simulink model "Appl_DrMemory_CtrlModel"  (R2018b)
settings: configuration reference "CodeConfig_10_ms" (kept outside this file)
undefined symbols (not defined in the file): CAL_DrMem_100MS, CAL_DrMem_90MS, D_DRMEM_SPEED_5, D_ToleranceDistance, FALSE, TRUE
libraries: DareLib x92, simulink x1
(part 2 of 3)

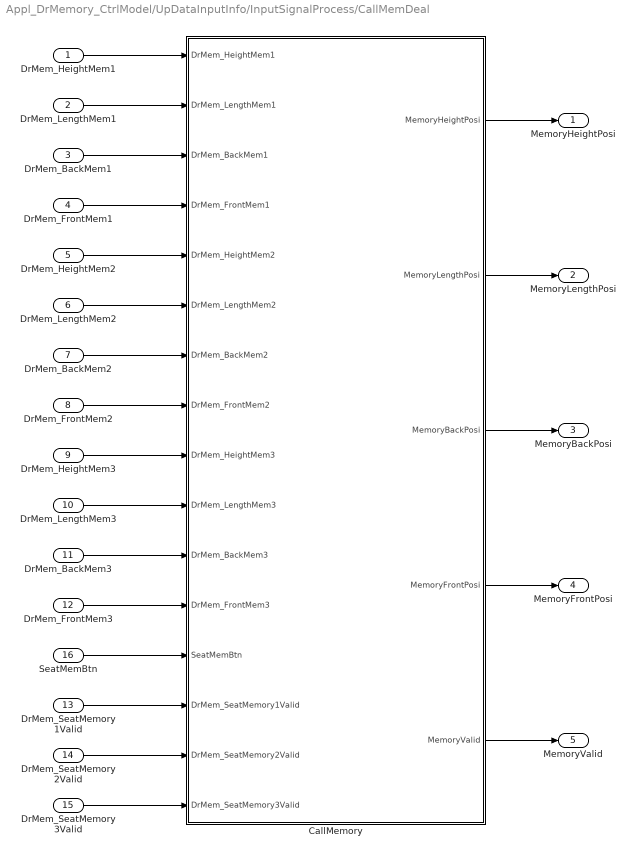
== system Appl_DrMemory_CtrlModel/UpDataInputInfo/InputSignalProcess/CallMemDeal ==
  DrMem_HeightMem1 : Inport
  DrMem_LengthMem1 : Inport  Port=2
  DrMem_BackMem1 : Inport  Port=3
  DrMem_FrontMem1 : Inport  Port=4
  DrMem_HeightMem2 : Inport  Port=5
  DrMem_LengthMem2 : Inport  Port=6
  DrMem_BackMem2 : Inport  Port=7
  DrMem_FrontMem2 : Inport  Port=8
  DrMem_HeightMem3 : Inport  Port=9
  DrMem_LengthMem3 : Inport  Port=10
  DrMem_BackMem3 : Inport  Port=11
  DrMem_FrontMem3 : Inport  Port=12
  DrMem_SeatMemory1Valid : Inport  Port=13
  DrMem_SeatMemory2Valid : Inport  Port=14
  DrMem_SeatMemory3Valid : Inport  Port=15
  SeatMemBtn : Inport  Port=16
  CallMemory : Stateflow chart  TreatAsAtomicUnit=on
  MemoryHeightPosi : Outport
  MemoryLengthPosi : Outport  Port=2
  MemoryBackPosi : Outport  Port=3
  MemoryFrontPosi : Outport  Port=4
  MemoryValid : Outport  Port=5
  wires:
  DrMem_LengthMem1/1 -> CallMemory/2(DrMem_LengthMem1)
  DrMem_BackMem1/1 -> CallMemory/3(DrMem_BackMem1)
  DrMem_HeightMem1/1 -> CallMemory/1(DrMem_HeightMem1)
  DrMem_FrontMem1/1 -> CallMemory/4(DrMem_FrontMem1)
  DrMem_HeightMem2/1 -> CallMemory/5(DrMem_HeightMem2)
  DrMem_LengthMem2/1 -> CallMemory/6(DrMem_LengthMem2)
  DrMem_BackMem2/1 -> CallMemory/7(DrMem_BackMem2)
  DrMem_FrontMem2/1 -> CallMemory/8(DrMem_FrontMem2)
  DrMem_HeightMem3/1 -> CallMemory/9(DrMem_HeightMem3)
  DrMem_LengthMem3/1 -> CallMemory/10(DrMem_LengthMem3)
  DrMem_BackMem3/1 -> CallMemory/11(DrMem_BackMem3)
  SeatMemBtn/1 -> CallMemory/13(SeatMemBtn)
  DrMem_FrontMem3/1 -> CallMemory/12(DrMem_FrontMem3)
  CallMemory/1(MemoryHeightPosi) -> MemoryHeightPosi/1
  CallMemory/3(MemoryBackPosi) -> MemoryBackPosi/1
  CallMemory/4(MemoryFrontPosi) -> MemoryFrontPosi/1
  CallMemory/2(MemoryLengthPosi) -> MemoryLengthPosi/1
  CallMemory/5(MemoryValid) -> MemoryValid/1
  DrMem_SeatMemory3Valid/1 -> CallMemory/16(DrMem_SeatMemory3Valid)
  DrMem_SeatMemory2Valid/1 -> CallMemory/15(DrMem_SeatMemory2Valid)
  DrMem_SeatMemory1Valid/1 -> CallMemory/14(DrMem_SeatMemory1Valid)

== system Appl_DrMemory_CtrlModel/UpDataInputInfo/InputSignalProcess/HmiMessageDeal ==
  DrMem_IVI_FLSeatMemSet1 : Inport
  DrMem_IVI_FLSeatMemSet2 : Inport  Port=2
  DrMem_IVI_FLSeatMemSet3 : Inport  Port=3
  HmiDeal : Stateflow chart  TreatAsAtomicUnit=on
  SeatMemBtn : Outport
  wires:
  DrMem_IVI_FLSeatMemSet1/1 -> HmiDeal/1(DrMem_IVI_FLSeatMemSet1)
  DrMem_IVI_FLSeatMemSet2/1 -> HmiDeal/2(DrMem_IVI_FLSeatMemSet2)
  HmiDeal/1(SeatMemBtn) -> SeatMemBtn/1
  DrMem_IVI_FLSeatMemSet3/1 -> HmiDeal/3(DrMem_IVI_FLSeatMemSet3)

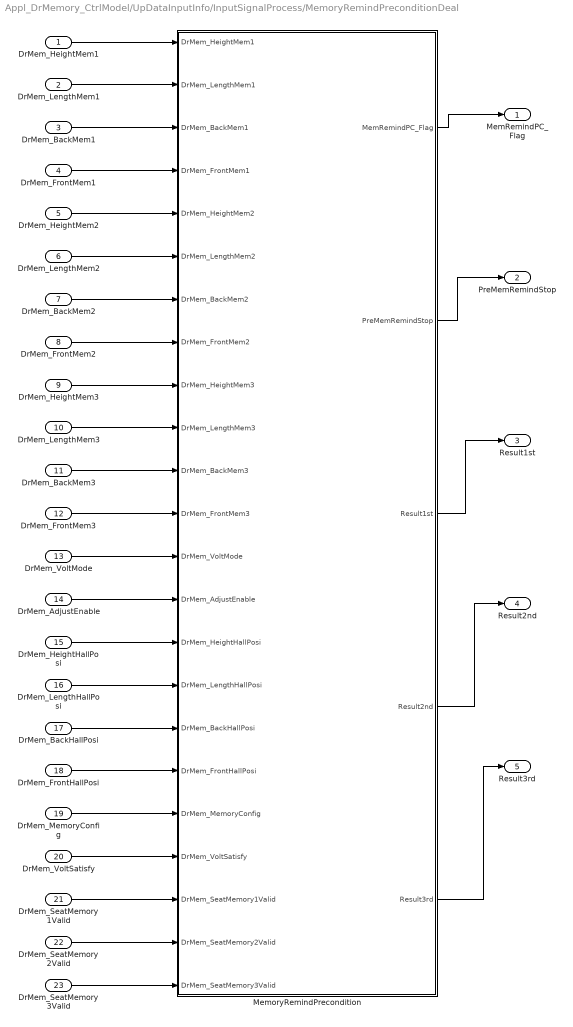
== system Appl_DrMemory_CtrlModel/UpDataInputInfo/InputSignalProcess/MemoryRemindPreconditionDeal ==
  DrMem_HeightMem1 : Inport
  DrMem_LengthMem1 : Inport  Port=2
  DrMem_BackMem1 : Inport  Port=3
  DrMem_FrontMem1 : Inport  Port=4
  DrMem_HeightMem2 : Inport  Port=5
  DrMem_LengthMem2 : Inport  Port=6
  DrMem_BackMem2 : Inport  Port=7
  DrMem_FrontMem2 : Inport  Port=8
  DrMem_HeightMem3 : Inport  Port=9
  DrMem_LengthMem3 : Inport  Port=10
  DrMem_BackMem3 : Inport  Port=11
  DrMem_FrontMem3 : Inport  Port=12
  DrMem_VoltMode : Inport  Port=13
  DrMem_AdjustEnable : Inport  Port=14
  DrMem_HeightHallPosi : Inport  Port=15
  DrMem_LengthHallPosi : Inport  Port=16
  DrMem_BackHallPosi : Inport  Port=17
  DrMem_FrontHallPosi : Inport  Port=18
  DrMem_MemoryConfig : Inport  Port=19
  DrMem_VoltSatisfy : Inport  Port=20
  DrMem_SeatMemory1Valid : Inport  Port=21
  DrMem_SeatMemory2Valid : Inport  Port=22
  DrMem_SeatMemory3Valid : Inport  Port=23
  MemoryRemindPrecondition : Stateflow chart  TreatAsAtomicUnit=on
  MemRemindPC_Flag : Outport
  PreMemRemindStop : Outport  Port=2
  Result1st : Outport  Port=3
  Result2nd : Outport  Port=4
  Result3rd : Outport  Port=5
  wires:
  DrMem_FrontMem3/1 -> MemoryRemindPrecondition/12(DrMem_FrontMem3)
  DrMem_VoltMode/1 -> MemoryRemindPrecondition/13(DrMem_VoltMode)
  DrMem_BackMem3/1 -> MemoryRemindPrecondition/11(DrMem_BackMem3)
  DrMem_LengthMem3/1 -> MemoryRemindPrecondition/10(DrMem_LengthMem3)
  DrMem_HeightMem3/1 -> MemoryRemindPrecondition/9(DrMem_HeightMem3)
  DrMem_FrontMem2/1 -> MemoryRemindPrecondition/8(DrMem_FrontMem2)
  DrMem_BackMem2/1 -> MemoryRemindPrecondition/7(DrMem_BackMem2)
  DrMem_LengthMem2/1 -> MemoryRemindPrecondition/6(DrMem_LengthMem2)
  DrMem_HeightMem2/1 -> MemoryRemindPrecondition/5(DrMem_HeightMem2)
  DrMem_FrontMem1/1 -> MemoryRemindPrecondition/4(DrMem_FrontMem1)
  DrMem_HeightMem1/1 -> MemoryRemindPrecondition/1(DrMem_HeightMem1)
  DrMem_BackMem1/1 -> MemoryRemindPrecondition/3(DrMem_BackMem1)
  DrMem_LengthMem1/1 -> MemoryRemindPrecondition/2(DrMem_LengthMem1)
  DrMem_AdjustEnable/1 -> MemoryRemindPrecondition/14(DrMem_AdjustEnable)
  DrMem_HeightHallPosi/1 -> MemoryRemindPrecondition/15(DrMem_HeightHallPosi)
  DrMem_LengthHallPosi/1 -> MemoryRemindPrecondition/16(DrMem_LengthHallPosi)
  DrMem_BackHallPosi/1 -> MemoryRemindPrecondition/17(DrMem_BackHallPosi)
  DrMem_FrontHallPosi/1 -> MemoryRemindPrecondition/18(DrMem_FrontHallPosi)
  MemoryRemindPrecondition/1(MemRemindPC_Flag) -> MemRemindPC_Flag/1
  MemoryRemindPrecondition/2(PreMemRemindStop) -> PreMemRemindStop/1
  MemoryRemindPrecondition/3(Result1st) -> Result1st/1
  MemoryRemindPrecondition/4(Result2nd) -> Result2nd/1
  MemoryRemindPrecondition/5(Result3rd) -> Result3rd/1
  DrMem_MemoryConfig/1 -> MemoryRemindPrecondition/19(DrMem_MemoryConfig)
  DrMem_VoltSatisfy/1 -> MemoryRemindPrecondition/20(DrMem_VoltSatisfy)
  DrMem_SeatMemory1Valid/1 -> MemoryRemindPrecondition/21(DrMem_SeatMemory1Valid)
  DrMem_SeatMemory3Valid/1 -> MemoryRemindPrecondition/23(DrMem_SeatMemory3Valid)
  DrMem_SeatMemory2Valid/1 -> MemoryRemindPrecondition/22(DrMem_SeatMemory2Valid)

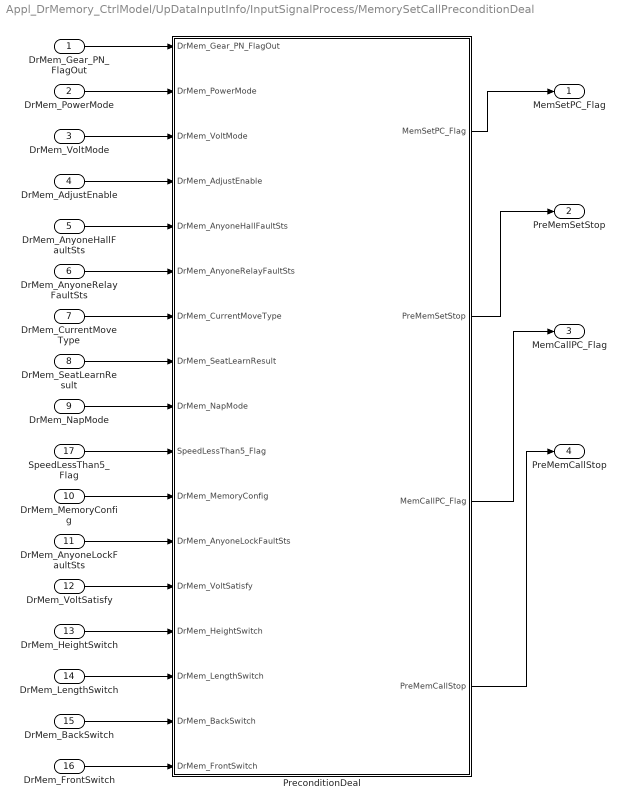
== system Appl_DrMemory_CtrlModel/UpDataInputInfo/InputSignalProcess/MemorySetCallPreconditionDeal ==
  DrMem_Gear_PN_FlagOut : Inport
  DrMem_PowerMode : Inport  Port=2
  DrMem_VoltMode : Inport  Port=3
  DrMem_AdjustEnable : Inport  Port=4
  DrMem_AnyoneHallFaultSts : Inport  Port=5
  DrMem_AnyoneRelayFaultSts : Inport  Port=6
  DrMem_CurrentMoveType : Inport  Port=7
  DrMem_SeatLearnResult : Inport  Port=8
  DrMem_NapMode : Inport  Port=9
  DrMem_MemoryConfig : Inport  Port=10
  DrMem_AnyoneLockFaultSts : Inport  Port=11
  DrMem_VoltSatisfy : Inport  Port=12
  DrMem_HeightSwitch : Inport  Port=13
  DrMem_LengthSwitch : Inport  Port=14
  DrMem_BackSwitch : Inport  Port=15
  DrMem_FrontSwitch : Inport  Port=16
  SpeedLessThan5_Flag : Inport  Port=17
  PreconditionDeal : Stateflow chart  TreatAsAtomicUnit=on
  MemSetPC_Flag : Outport
  PreMemSetStop : Outport  Port=2
  MemCallPC_Flag : Outport  Port=3
  PreMemCallStop : Outport  Port=4
  wires:
  DrMem_Gear_PN_FlagOut/1 -> PreconditionDeal/1(DrMem_Gear_PN_FlagOut)
  DrMem_PowerMode/1 -> PreconditionDeal/2(DrMem_PowerMode)
  DrMem_VoltMode/1 -> PreconditionDeal/3(DrMem_VoltMode)
  DrMem_AdjustEnable/1 -> PreconditionDeal/4(DrMem_AdjustEnable)
  DrMem_AnyoneHallFaultSts/1 -> PreconditionDeal/5(DrMem_AnyoneHallFaultSts)
  DrMem_CurrentMoveType/1 -> PreconditionDeal/7(DrMem_CurrentMoveType)
  DrMem_SeatLearnResult/1 -> PreconditionDeal/8(DrMem_SeatLearnResult)
  DrMem_NapMode/1 -> PreconditionDeal/9(DrMem_NapMode)
  SpeedLessThan5_Flag/1 -> PreconditionDeal/10(SpeedLessThan5_Flag)
  DrMem_AnyoneRelayFaultSts/1 -> PreconditionDeal/6(DrMem_AnyoneRelayFaultSts)
  PreconditionDeal/1(MemSetPC_Flag) -> MemSetPC_Flag/1
  PreconditionDeal/2(PreMemSetStop) -> PreMemSetStop/1
  PreconditionDeal/3(MemCallPC_Flag) -> MemCallPC_Flag/1
  PreconditionDeal/4(PreMemCallStop) -> PreMemCallStop/1
  DrMem_MemoryConfig/1 -> PreconditionDeal/11(DrMem_MemoryConfig)
  DrMem_AnyoneLockFaultSts/1 -> PreconditionDeal/12(DrMem_AnyoneLockFaultSts)
  DrMem_VoltSatisfy/1 -> PreconditionDeal/13(DrMem_VoltSatisfy)
  DrMem_HeightSwitch/1 -> PreconditionDeal/14(DrMem_HeightSwitch)
  DrMem_LengthSwitch/1 -> PreconditionDeal/15(DrMem_LengthSwitch)
  DrMem_BackSwitch/1 -> PreconditionDeal/16(DrMem_BackSwitch)
  DrMem_FrontSwitch/1 -> PreconditionDeal/17(DrMem_FrontSwitch)

== system Appl_DrMemory_CtrlModel/UpDataInputInfo/InputSignalProcess/VehicleSpeedDeal ==
  DrMem_0x284_SpeedLostFlag : Inport
  DrMem_VehicleSpeedValid : Inport  Port=2
  DrMem_VehicleSpeed : Inport  Port=3
  SpeedDeal : Stateflow chart  TreatAsAtomicUnit=on
  "SpeedLessThan5_Flag " : Outport
  wires:
  SpeedDeal/1(SpeedLessThan5_Flag) -> "SpeedLessThan5_Flag "/1
  DrMem_0x284_SpeedLostFlag/1 -> SpeedDeal/1(DrMem_0x284_SpeedLostFlag)
  DrMem_VehicleSpeedValid/1 -> SpeedDeal/2(DrMem_VehicleSpeedValid)
  DrMem_VehicleSpeed/1 -> SpeedDeal/3(DrMem_VehicleSpeed)

== system Appl_DrMemory_CtrlModel/LogicCtrl/LocalAdjustCtrl/MemorySetLogic/FirstPosiMemSetFunc/FirstPosiMemSetFunc/MemoryBack ==
  CurrentB : Inport
  f : TriggerPort  TriggerType=function-call  VariantControl=(inherit)
      settings: CopyFcn=Stateflow.SLINSF.SimulinkMan.removeBlockPreDeleteFcn  PreDeleteFcn=Stateflow.SLINSF.SimulinkMan.unsafePredeleteFcn
  WelcomeRunStatus : DareLib/Dare/setAPI_type  g_funcname=Srvl_SetMemIndexDataU16  g_param=EN_MemIndex_DrMem1_Back  g_type=uint16  g_size=-1
      settings: AttributesFormatString=%<g_funcname>  SourceProductName=Dare Library
  wires:
  CurrentB/1 -> WelcomeRunStatus/1

== system Appl_DrMemory_CtrlModel/LogicCtrl/LocalAdjustCtrl/MemorySetLogic/FirstPosiMemSetFunc/FirstPosiMemSetFunc/MemoryFront ==
  CurrentF : Inport
  f : TriggerPort  TriggerType=function-call  VariantControl=(inherit)
      settings: CopyFcn=Stateflow.SLINSF.SimulinkMan.removeBlockPreDeleteFcn  PreDeleteFcn=Stateflow.SLINSF.SimulinkMan.unsafePredeleteFcn
  WelcomeRunStatus : DareLib/Dare/setAPI_type  g_funcname=Srvl_SetMemIndexDataU16  g_param=EN_MemIndex_DrMem1_Front  g_type=uint16  g_size=-1
      settings: AttributesFormatString=%<g_funcname>  SourceProductName=Dare Library
  wires:
  CurrentF/1 -> WelcomeRunStatus/1

== system Appl_DrMemory_CtrlModel/LogicCtrl/LocalAdjustCtrl/MemorySetLogic/FirstPosiMemSetFunc/FirstPosiMemSetFunc/MemoryHight ==
  CurrentH : Inport
  f : TriggerPort  TriggerType=function-call  VariantControl=(inherit)
      settings: CopyFcn=Stateflow.SLINSF.SimulinkMan.removeBlockPreDeleteFcn  PreDeleteFcn=Stateflow.SLINSF.SimulinkMan.unsafePredeleteFcn
  WelcomeRunStatus : DareLib/Dare/setAPI_type  g_funcname=Srvl_SetMemIndexDataU16  g_param=EN_MemIndex_DrMem1_Height  g_type=uint16  g_size=-1
      settings: AttributesFormatString=%<g_funcname>  SourceProductName=Dare Library
  wires:
  CurrentH/1 -> WelcomeRunStatus/1

== system Appl_DrMemory_CtrlModel/LogicCtrl/LocalAdjustCtrl/MemorySetLogic/FirstPosiMemSetFunc/FirstPosiMemSetFunc/MemoryLength ==
  CurrentL : Inport
  f : TriggerPort  TriggerType=function-call  VariantControl=(inherit)
      settings: CopyFcn=Stateflow.SLINSF.SimulinkMan.removeBlockPreDeleteFcn  PreDeleteFcn=Stateflow.SLINSF.SimulinkMan.unsafePredeleteFcn
  WelcomeRunStatus : DareLib/Dare/setAPI_type  g_funcname=Srvl_SetMemIndexDataU16  g_param=EN_MemIndex_DrMem1_Length  g_type=uint16  g_size=-1
      settings: AttributesFormatString=%<g_funcname>  SourceProductName=Dare Library
  wires:
  CurrentL/1 -> WelcomeRunStatus/1

== system Appl_DrMemory_CtrlModel/LogicCtrl/LocalAdjustCtrl/MemorySetLogic/FirstPosiMemSetFunc/FirstPosiMemSetFunc/MemoryValid ==
  Sts : Inport
  f : TriggerPort  TriggerType=function-call  VariantControl=(inherit)
      settings: CopyFcn=Stateflow.SLINSF.SimulinkMan.removeBlockPreDeleteFcn  PreDeleteFcn=Stateflow.SLINSF.SimulinkMan.unsafePredeleteFcn
  WelcomeRunStatus : DareLib/Dare/setAPI_type  g_funcname=Srvl_SetMemIndexDataU8  g_param=EN_MemIndex_DrMem1_ValidFlag  g_type=uint16  g_size=-1
      settings: AttributesFormatString=%<g_funcname>  SourceProductName=Dare Library
  wires:
  Sts/1 -> WelcomeRunStatus/1

== system Appl_DrMemory_CtrlModel/LogicCtrl/LocalAdjustCtrl/MemorySetLogic/SecondPosiMemSetFunc/SecondPosiMemSetFunc/MemoryBack ==
  CurrentB : Inport
  f : TriggerPort  TriggerType=function-call  VariantControl=(inherit)
      settings: CopyFcn=Stateflow.SLINSF.SimulinkMan.removeBlockPreDeleteFcn  PreDeleteFcn=Stateflow.SLINSF.SimulinkMan.unsafePredeleteFcn
  WelcomeRunStatus : DareLib/Dare/setAPI_type  g_funcname=Srvl_SetMemIndexDataU16  g_param=EN_MemIndex_DrMem2_Back  g_type=uint16  g_size=-1
      settings: AttributesFormatString=%<g_funcname>  SourceProductName=Dare Library
  wires:
  CurrentB/1 -> WelcomeRunStatus/1

== system Appl_DrMemory_CtrlModel/LogicCtrl/LocalAdjustCtrl/MemorySetLogic/SecondPosiMemSetFunc/SecondPosiMemSetFunc/MemoryFront ==
  CurrentF : Inport
  f : TriggerPort  TriggerType=function-call  VariantControl=(inherit)
      settings: CopyFcn=Stateflow.SLINSF.SimulinkMan.removeBlockPreDeleteFcn  PreDeleteFcn=Stateflow.SLINSF.SimulinkMan.unsafePredeleteFcn
  WelcomeRunStatus : DareLib/Dare/setAPI_type  g_funcname=Srvl_SetMemIndexDataU16  g_param=EN_MemIndex_DrMem2_Front  g_type=uint16  g_size=-1
      settings: AttributesFormatString=%<g_funcname>  SourceProductName=Dare Library
  wires:
  CurrentF/1 -> WelcomeRunStatus/1

== system Appl_DrMemory_CtrlModel/LogicCtrl/LocalAdjustCtrl/MemorySetLogic/SecondPosiMemSetFunc/SecondPosiMemSetFunc/MemoryHight ==
  CurrentH : Inport
  f : TriggerPort  TriggerType=function-call  VariantControl=(inherit)
      settings: CopyFcn=Stateflow.SLINSF.SimulinkMan.removeBlockPreDeleteFcn  PreDeleteFcn=Stateflow.SLINSF.SimulinkMan.unsafePredeleteFcn
  WelcomeRunStatus : DareLib/Dare/setAPI_type  g_funcname=Srvl_SetMemIndexDataU16  g_param=EN_MemIndex_DrMem2_Height  g_type=uint16  g_size=-1
      settings: AttributesFormatString=%<g_funcname>  SourceProductName=Dare Library
  wires:
  CurrentH/1 -> WelcomeRunStatus/1

== system Appl_DrMemory_CtrlModel/LogicCtrl/LocalAdjustCtrl/MemorySetLogic/SecondPosiMemSetFunc/SecondPosiMemSetFunc/MemoryLength ==
  CurrentL : Inport
  f : TriggerPort  TriggerType=function-call  VariantControl=(inherit)
      settings: CopyFcn=Stateflow.SLINSF.SimulinkMan.removeBlockPreDeleteFcn  PreDeleteFcn=Stateflow.SLINSF.SimulinkMan.unsafePredeleteFcn
  WelcomeRunStatus : DareLib/Dare/setAPI_type  g_funcname=Srvl_SetMemIndexDataU16  g_param=EN_MemIndex_DrMem2_Length  g_type=uint16  g_size=-1
      settings: AttributesFormatString=%<g_funcname>  SourceProductName=Dare Library
  wires:
  CurrentL/1 -> WelcomeRunStatus/1

== system Appl_DrMemory_CtrlModel/LogicCtrl/LocalAdjustCtrl/MemorySetLogic/SecondPosiMemSetFunc/SecondPosiMemSetFunc/MemoryValid ==
  Sts : Inport
  f : TriggerPort  TriggerType=function-call  VariantControl=(inherit)
      settings: CopyFcn=Stateflow.SLINSF.SimulinkMan.removeBlockPreDeleteFcn  PreDeleteFcn=Stateflow.SLINSF.SimulinkMan.unsafePredeleteFcn
  WelcomeRunStatus : DareLib/Dare/setAPI_type  g_funcname=Srvl_SetMemIndexDataU8  g_param=EN_MemIndex_DrMem2_ValidFlag  g_type=uint16  g_size=-1
      settings: AttributesFormatString=%<g_funcname>  SourceProductName=Dare Library
  wires:
  Sts/1 -> WelcomeRunStatus/1

== system Appl_DrMemory_CtrlModel/LogicCtrl/LocalAdjustCtrl/MemorySetLogic/ThirdPosiMemSetFunc/ThirdPosiMemSetFunc/MemoryBack ==
  CurrentB : Inport
  f : TriggerPort  TriggerType=function-call  VariantControl=(inherit)
      settings: CopyFcn=Stateflow.SLINSF.SimulinkMan.removeBlockPreDeleteFcn  PreDeleteFcn=Stateflow.SLINSF.SimulinkMan.unsafePredeleteFcn
  WelcomeRunStatus : DareLib/Dare/setAPI_type  g_funcname=Srvl_SetMemIndexDataU16  g_param=EN_MemIndex_DrMem3_Back  g_type=uint16  g_size=-1
      settings: AttributesFormatString=%<g_funcname>  SourceProductName=Dare Library
  wires:
  CurrentB/1 -> WelcomeRunStatus/1

== system Appl_DrMemory_CtrlModel/LogicCtrl/LocalAdjustCtrl/MemorySetLogic/ThirdPosiMemSetFunc/ThirdPosiMemSetFunc/MemoryFront ==
  CurrentF : Inport
  f : TriggerPort  TriggerType=function-call  VariantControl=(inherit)
      settings: CopyFcn=Stateflow.SLINSF.SimulinkMan.removeBlockPreDeleteFcn  PreDeleteFcn=Stateflow.SLINSF.SimulinkMan.unsafePredeleteFcn
  WelcomeRunStatus : DareLib/Dare/setAPI_type  g_funcname=Srvl_SetMemIndexDataU16  g_param=EN_MemIndex_DrMem3_Front  g_type=uint16  g_size=-1
      settings: AttributesFormatString=%<g_funcname>  SourceProductName=Dare Library
  wires:
  CurrentF/1 -> WelcomeRunStatus/1

== system Appl_DrMemory_CtrlModel/LogicCtrl/LocalAdjustCtrl/MemorySetLogic/ThirdPosiMemSetFunc/ThirdPosiMemSetFunc/MemoryHight ==
  CurrentH : Inport
  f : TriggerPort  TriggerType=function-call  VariantControl=(inherit)
      settings: CopyFcn=Stateflow.SLINSF.SimulinkMan.removeBlockPreDeleteFcn  PreDeleteFcn=Stateflow.SLINSF.SimulinkMan.unsafePredeleteFcn
  WelcomeRunStatus : DareLib/Dare/setAPI_type  g_funcname=Srvl_SetMemIndexDataU16  g_param=EN_MemIndex_DrMem3_Height  g_type=uint16  g_size=-1
      settings: AttributesFormatString=%<g_funcname>  SourceProductName=Dare Library
  wires:
  CurrentH/1 -> WelcomeRunStatus/1

== system Appl_DrMemory_CtrlModel/LogicCtrl/LocalAdjustCtrl/MemorySetLogic/ThirdPosiMemSetFunc/ThirdPosiMemSetFunc/MemoryLength ==
  CurrentL : Inport
  f : TriggerPort  TriggerType=function-call  VariantControl=(inherit)
      settings: CopyFcn=Stateflow.SLINSF.SimulinkMan.removeBlockPreDeleteFcn  PreDeleteFcn=Stateflow.SLINSF.SimulinkMan.unsafePredeleteFcn
  WelcomeRunStatus : DareLib/Dare/setAPI_type  g_funcname=Srvl_SetMemIndexDataU16  g_param=EN_MemIndex_DrMem3_Length  g_type=uint16  g_size=-1
      settings: AttributesFormatString=%<g_funcname>  SourceProductName=Dare Library
  wires:
  CurrentL/1 -> WelcomeRunStatus/1

== system Appl_DrMemory_CtrlModel/LogicCtrl/LocalAdjustCtrl/MemorySetLogic/ThirdPosiMemSetFunc/ThirdPosiMemSetFunc/MemoryValid ==
  Sts : Inport
  f : TriggerPort  TriggerType=function-call  VariantControl=(inherit)
      settings: CopyFcn=Stateflow.SLINSF.SimulinkMan.removeBlockPreDeleteFcn  PreDeleteFcn=Stateflow.SLINSF.SimulinkMan.unsafePredeleteFcn
  WelcomeRunStatus : DareLib/Dare/setAPI_type  g_funcname=Srvl_SetMemIndexDataU8  g_param=EN_MemIndex_DrMem3_ValidFlag  g_type=uint16  g_size=-1
      settings: AttributesFormatString=%<g_funcname>  SourceProductName=Dare Library
  wires:
  Sts/1 -> WelcomeRunStatus/1

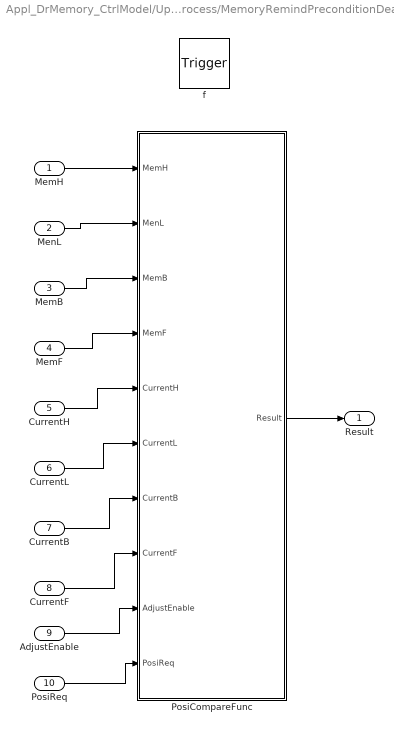
== system Appl_DrMemory_CtrlModel/UpDataInputInfo/InputSignalProcess/MemoryRemindPreconditionDeal/MemoryRemindPrecondition/PosiCompareFunc ==
  MemH : Inport
  MenL : Inport  Port=2
  MemB : Inport  Port=3
  MemF : Inport  Port=4
  CurrentH : Inport  Port=5
  CurrentL : Inport  Port=6
  CurrentB : Inport  Port=7
  CurrentF : Inport  Port=8
  AdjustEnable : Inport  Port=9
  PosiReq : Inport  Port=10
  f : TriggerPort  TriggerType=function-call  VariantControl=(inherit)
      settings: CopyFcn=Stateflow.SLINSF.SimulinkMan.removeBlockPreDeleteFcn  PreDeleteFcn=Stateflow.SLINSF.SimulinkMan.unsafePredeleteFcn
  PosiCompareFunc : Stateflow chart  TreatAsAtomicUnit=on
  "Result " : Outport
  wires:
  MemB/1 -> PosiCompareFunc/3(MemB)
  MemF/1 -> PosiCompareFunc/4(MemF)
  CurrentH/1 -> PosiCompareFunc/5(CurrentH)
  MenL/1 -> PosiCompareFunc/2(MenL)
  CurrentL/1 -> PosiCompareFunc/6(CurrentL)
  MemH/1 -> PosiCompareFunc/1(MemH)
  CurrentB/1 -> PosiCompareFunc/7(CurrentB)
  CurrentF/1 -> PosiCompareFunc/8(CurrentF)
  PosiCompareFunc/1(Result) -> "Result "/1
  AdjustEnable/1 -> PosiCompareFunc/9(AdjustEnable)
  PosiReq/1 -> PosiCompareFunc/10(PosiReq)

== stateflow chart Appl_DrMemory_CtrlModel/UpDataInputInfo/InputSignalProcess/CallMemDeal/CallMemory ==
  state NoneMemoryCall
    en:
    MemoryHeightPosi = 0;
    MemoryLengthPosi = 0;
    MemoryBackPosi = 0;
    MemoryFrontPosi = 0;
    MemoryValid = FALSE;
  state AcquireMemory2ndPosi
    en:
    MemoryHeightPosi = DrMem_HeightMem2;
    MemoryLengthPosi = DrMem_LengthMem2;
    MemoryBackPosi = DrMem_BackMem2;
    MemoryFrontPosi = DrMem_FrontMem2;
    MemoryValid = DrMem_SeatMemory2Valid;
  state AcquireMemory1stPosi
    en:
    MemoryHeightPosi = DrMem_HeightMem1;
    MemoryLengthPosi = DrMem_LengthMem1;
    MemoryBackPosi = DrMem_BackMem1;
    MemoryFrontPosi = DrMem_FrontMem1;
    MemoryValid = DrMem_SeatMemory1Valid;
  state AcquireMemory3rdPosi
    en:
    MemoryHeightPosi = DrMem_HeightMem3;
    MemoryLengthPosi = DrMem_LengthMem3;
    MemoryBackPosi = DrMem_BackMem3;
    MemoryFrontPosi = DrMem_FrontMem3;
    MemoryValid = DrMem_SeatMemory3Valid;
  (default) -> NoneMemoryCall
  NoneMemoryCall -> AcquireMemory1stPosi [order 1] : /* 调用位置1 */
      | [SeatMemBtn == enMemBtn.EN_MemBtn_Call1]
  AcquireMemory1stPosi -> NoneMemoryCall [order 1] : /* 无调用 */
      | [SeatMemBtn != enMemBtn.EN_MemBtn_Call1 ...
      | && SeatMemBtn != enMemBtn.EN_MemBtn_Call2 ...
      | && SeatMemBtn != enMemBtn.EN_MemBtn_Call3]
  NoneMemoryCall -> AcquireMemory2ndPosi [order 2] : /* 调用位置2 */
      | [SeatMemBtn == enMemBtn.EN_MemBtn_Call2]
  AcquireMemory2ndPosi -> NoneMemoryCall [order 1] : /* 无调用 */
      | [SeatMemBtn != enMemBtn.EN_MemBtn_Call1 ...
      | && SeatMemBtn != enMemBtn.EN_MemBtn_Call2 ...
      | && SeatMemBtn != enMemBtn.EN_MemBtn_Call3]
  NoneMemoryCall -> AcquireMemory3rdPosi [order 3] : /* 调用位置3 */
      | [SeatMemBtn == enMemBtn.EN_MemBtn_Call3]
  AcquireMemory3rdPosi -> NoneMemoryCall [order 1] : /* 无调用 */
      | [SeatMemBtn != enMemBtn.EN_MemBtn_Call1 ...
      | && SeatMemBtn != enMemBtn.EN_MemBtn_Call2 ...
      | && SeatMemBtn != enMemBtn.EN_MemBtn_Call3]
  AcquireMemory1stPosi -> AcquireMemory2ndPosi [order 3] : /* 调用位置2 */
      | [SeatMemBtn == enMemBtn.EN_MemBtn_Call2]
  AcquireMemory3rdPosi -> AcquireMemory2ndPosi [order 3] : /* 调用位置2 */
      | [SeatMemBtn == enMemBtn.EN_MemBtn_Call2]
  AcquireMemory2ndPosi -> AcquireMemory3rdPosi [order 3] : /* 调用位置3 */
      | [SeatMemBtn == enMemBtn.EN_MemBtn_Call3]
  AcquireMemory2ndPosi -> AcquireMemory1stPosi [order 2] : /* 调用位置1 */
      | [SeatMemBtn == enMemBtn.EN_MemBtn_Call1]
  AcquireMemory1stPosi -> AcquireMemory3rdPosi [order 2] : /* 调用位置3 */
      | [SeatMemBtn == enMemBtn.EN_MemBtn_Call3]
  AcquireMemory3rdPosi -> AcquireMemory1stPosi [order 2] : /* 调用位置1 */
      | [SeatMemBtn == enMemBtn.EN_MemBtn_Call1]
  data: DrMem_HeightMem1 input; MemoryHeightPosi output uint16; MemoryLengthPosi output uint16; MemoryBackPosi output uint16; MemoryFrontPosi output uint16; MemoryValid output uint8; DrMem_LengthMem1 input; DrMem_BackMem1 input; DrMem_FrontMem1 input; DrMem_HeightMem2 input; DrMem_LengthMem2 input; DrMem_BackMem2 input; DrMem_FrontMem2 input; DrMem_HeightMem3 input; DrMem_LengthMem3 input; DrMem_BackMem3 input; DrMem_FrontMem3 input; SeatMemBtn input; TRUE parameter; FALSE parameter; DrMem_SeatMemory1Valid input; DrMem_SeatMemory2Valid input; DrMem_SeatMemory3Valid input

== stateflow chart Appl_DrMemory_CtrlModel/UpDataInputInfo/InputSignalProcess/MemoryRemindPreconditionDeal/MemoryRemindPrecondition ==
  state Result = PosiCompareFunc(MemH,MenL,MemB,MemF,CurrentH,CurrentL,CurrentB,CurrentF,AdjustEnable,PosiReq) [function]
  state CompareCurrentAndMemoryPosi [parallel]
    du:
    Result1st = PosiCompareFunc(DrMem_HeightMem1,DrMem_LengthMem1,DrMem_BackMem1,DrMem_FrontMem1,DrMem_HeightHallPosi,DrMem_LengthHallPosi,DrMem_BackHallPosi,DrMem_FrontHallPosi,DrMem_AdjustEnable,DrMem_SeatMemory1Valid);
    Result2nd = PosiCompareFunc(DrMem_HeightMem2,DrMem_LengthMem2,DrMem_BackMem2,DrMem_FrontMem2,DrMem_HeightHallPosi,DrMem_LengthHallPosi,DrMem_BackHallPosi,DrMem_FrontHallPosi,DrMem_AdjustEnable,DrMem_SeatMemory2Valid);
    Result3rd = PosiCompareFunc(DrMem_HeightMem3,DrMem_LengthMem3,DrMem_BackMem3,DrMem_FrontMem3,DrMem_HeightHallPosi,DrMem_LengthHallPosi,DrMem_BackHallPosi,DrMem_FrontHallPosi,DrMem_AdjustEnable,DrMem_SeatMemory3Valid);
    settings: executionOrder=1
  state MemoryRemindPreconditionDeal [parallel]
    settings: executionOrder=2
    state PreconditionNotSatisfied
      en:
      MemRemindPC_Flag = FALSE;
    state PreconditionSatisfied
      en:
      MemRemindPC_Flag = TRUE;
    (default) -> PreconditionNotSatisfied
    PreconditionNotSatisfied -> PreconditionSatisfied : /*主驾调节配置 == 1 或者 == 2
        | &&记忆功能使能 == 0x1:TRUE
        | && 记忆提示功能使能 == 0x1:Enable
        | && 电压模式 == 正常
        | /PreMemRemindStop = 0x0:enNone;*/
        | [(DrMem_AdjustEnable == 1 || DrMem_AdjustEnable == 2)...
        | && DrMem_MemoryConfig == TRUE ...
        | && DrMem_VoltSatisfy == TRUE ...
        | && DrMem_VoltMode == enFinalPowerMode.EN_NORMAL_VOLT]
        | /PreMemRemindStop = enMemStopCause.EN_MemStop_NULL;
    PreconditionSatisfied -> PreconditionNotSatisfied [order 1] : /*主驾调节配置 != 1 且 != 2
        | || F101记忆功能 != 0x1:TRUE
        | || 记忆提示功能配置 != 0x1:Enable
        | /PreMemRemindStop = 0xA:enConfigError;*/
        | [DrMem_MemoryConfig != TRUE ...
        | ||(DrMem_AdjustEnable != 1 && DrMem_AdjustEnable != 2)]
        | /PreMemRemindStop = enMemStopCause.EN_MemStop_ConfigError;
    PreconditionSatisfied -> PreconditionNotSatisfied [order 2] : /*电压模式 != 正常
        | /PreMemRemindStop = 0xE:enVoltageError;*/
        | [DrMem_VoltMode != enFinalPowerMode.EN_NORMAL_VOLT ...
        | || DrMem_VoltSatisfy != TRUE]
        | /PreMemRemindStop = enMemStopCause.EN_MemStop_VoltageErr;
  data: MemH function_input; MenL function_input; MemB function_input; MemF function_input; CurrentH function_input; CurrentL function_input; CurrentB function_input; CurrentF function_input; Result function_output; AdjustEnable function_input; PosiReq function_input; DrMem_HeightMem1 input; DrMem_LengthMem1 input; DrMem_BackMem1 input; DrMem_FrontMem1 input; DrMem_HeightMem2 input; DrMem_LengthMem2 input; DrMem_BackMem2 input; DrMem_FrontMem2 input; DrMem_HeightMem3 input; DrMem_LengthMem3 input; DrMem_BackMem3 input; DrMem_FrontMem3 input; DrMem_VoltMode input; TRUE parameter; DrMem_AdjustEnable input; FALSE parameter; MemRemindPC_Flag output uint8; PreMemRemindStop output Enum: enMemStopCause; Result1st output uint8; Result2nd output uint8; Result3rd output uint8; DrMem_HeightHallPosi input; DrMem_LengthHallPosi input; DrMem_BackHallPosi input; DrMem_FrontHallPosi input; DrMem_MemoryConfig input; DrMem_VoltSatisfy input; DrMem_SeatMemory1Valid input; DrMem_SeatMemory2Valid input; DrMem_SeatMemory3Valid input

== stateflow chart Appl_DrMemory_CtrlModel/LogicCtrl/LocalAdjustCtrl/MemorySetLogic ==
  state FirstPosiMemSetFunc(SeatMemCfg,CurrentH,CurrentL,CurrentB,CurrentF) [function]
  state MemorySetInactive
    en:
    FLSeatMemSetSts = enMemSetFb.EN_MemSetFb_NULL;
    MsgSendFinishedFlag = FALSE;
  state SecondPosiMemSetFunc(SeatMemCfg,CurrentH,CurrentL,CurrentB,CurrentF) [function]
  state MemorySetActive
    state Wait
      (default) -> (junction 127)
      Wait -> (junction 127) [order 1]
      (junction 127) -> (junction 30)
      (junction 30) -> (junction 122) [order 1] : /*初始前置条件不符合*/
          | [MemSetPC_Flag == FALSE]
      (junction 30) -> (junction 33) [order 2]
      (junction 122) -> (junction 124) : {WaitTimer = 0;}
      (junction 33) -> (junction 35) [order 1] : /*记忆设置1*/
          | [SeatMemBtn == enMemBtn.EN_MemBtn_Set1]
      (junction 33) -> (junction 39) [order 2]
      (junction 35) -> (junction 37) : {FLTempSeatMemSetSts = enMemSetFb.EN_MemSetFb_S1;
          | FirstPosiMemSetFunc(DrMem_AdjustEnable,DrMem_HeightHallPosi,DrMem_LengthHallPosi,DrMem_BackHallPosi,DrMem_FrontHallPosi);}
      (junction 37) -> (junction 39)
      (junction 39) -> (junction 42)
      (junction 42) -> (junction 44) [order 1] : /*记忆设置2*/
          | [SeatMemBtn == enMemBtn.EN_MemBtn_Set2]
      (junction 42) -> (junction 48) [order 2]
      (junction 44) -> (junction 46) : {FLTempSeatMemSetSts = enMemSetFb.EN_MemSetFb_S2;
          | SecondPosiMemSetFunc(DrMem_AdjustEnable,DrMem_HeightHallPosi,DrMem_LengthHallPosi,DrMem_BackHallPosi,DrMem_FrontHallPosi);}
      (junction 46) -> (junction 48)
      (junction 48) -> (junction 51)
      (junction 51) -> (junction 53) [order 1] : /*记忆设置3*/
          | [SeatMemBtn == enMemBtn.EN_MemBtn_Set3]
      (junction 51) -> (junction 57) [order 2]
      (junction 53) -> (junction 55) : {FLTempSeatMemSetSts = enMemSetFb.EN_MemSetFb_S3;
          | ThirdPosiMemSetFunc(DrMem_AdjustEnable,DrMem_HeightHallPosi,DrMem_LengthHallPosi,DrMem_BackHallPosi,DrMem_FrontHallPosi);}
      (junction 55) -> (junction 57)
      (junction 57) -> (junction 60) : {FLSeatMemSetSts = enMemSetFb.EN_MemSetFb_NULL;}
      (junction 60) -> (junction 62)
      (junction 62) -> (junction 64) [order 1] : /*使用延时代替EEPROM操作结果*/
          | [WaitTimer < CAL_DrMem_100MS]
      (junction 62) -> (junction 68) [order 2] : {WaitTimer = CAL_DrMem_100MS;}
      (junction 64) -> (junction 66) : {WaitTimer++ ;}
      (junction 66) -> (junction 68)
      (junction 124) -> (junction 66)
      (junction 68) -> (junction 72)
    state Succeed
      en:
      FLSeatMemSetSts = FLTempSeatMemSetSts;
      WaitTimer = 0;
      WaitTimeCnt = 0;
      SetCanSendFLSeatMemSts(FLSeatMemSetSts);
      SetCanSendEvent();
      du:
      WaitTimeCnt += 1;
    state Fail
      en:
      FLSeatMemSetSts = enMemSetFb.EN_MemSetFb_Fail;
      WaitTimer = 0;
      WaitTimeCnt = 0;
      SetCanSendFLSeatMemSts(FLSeatMemSetSts);
      SetCanSendEvent();
      du:
      WaitTimeCnt += 1;
    note: /*如果服务层没有CAN反馈标志，使用延时90ms(20ms/5帧)*/
    state MessageSendFinish
      en:
      MsgSendFinishedFlag = TRUE;
      FLSeatMemSetSts = enMemSetFb.EN_MemSetFb_NULL;
    (default) -> Wait
    Wait -> Succeed [order 2] : /*存储结束*/
        | [WaitTimer >= CAL_DrMem_100MS]
    Wait -> Fail [order 1] : /*前置条件不符合*/
        | [MemSetPC_Flag == FALSE]
        | /MemSetStopReason = PreMemSetStop;
    Wait -> Fail [commented out] : /*记忆存储失败，如果无此接口，删除*/
    Succeed -> MessageSendFinish : /*Srvl_CAN反馈报文发送完成 || 延时90ms*/
        | [WaitTimeCnt >= CAL_DrMem_90MS || GetCanSendEvent() == TRUE]
    Fail -> MessageSendFinish : /*Srvl_CAN反馈报文发送完成 || 延时90ms*/
        | [WaitTimeCnt >= CAL_DrMem_90MS || GetCanSendEvent() == TRUE]
  state ThirdPosiMemSetFunc(SeatMemCfg,CurrentH,CurrentL,CurrentB,CurrentF) [function]
  state SetCanSendEvent [function]
  state Out1 = GetCanSendEvent [function]
  state SetCanSendFLSeatMemSts(In1) [function]
  (default) -> MemorySetInactive
  MemorySetInactive -> MemorySetActive [order 1] : /*SeatMemBtn变为MemorizeButton1*/
      | [hasChangedTo(SeatMemBtn,enMemBtn.EN_MemBtn_Set1)]
  MemorySetInactive -> MemorySetActive [order 2] : /*SeatMemBtn变为MemorizeButton2*/
      | [hasChangedTo(SeatMemBtn,enMemBtn.EN_MemBtn_Set2)]
  MemorySetInactive -> MemorySetActive [order 3] : /*SeatMemBtn变为MemorizeButton3*/
      | [hasChangedTo(SeatMemBtn,enMemBtn.EN_MemBtn_Set3)]
  MemorySetActive -> MemorySetInactive : [MsgSendFinishedFlag == TRUE]
  data: SeatMemCfg function_input; CurrentH function_input; CurrentL function_input; CurrentB function_input; CurrentF function_input; SeatMemCfg function_input; CurrentH function_input; CurrentL function_input; CurrentB function_input; CurrentF function_input; SeatMemCfg function_input; CurrentH function_input; CurrentL function_input; CurrentB function_input; CurrentF function_input; Out1 function_output; In1 function_input; FLSeatMemSetSts output Enum: enMemSetFb; MsgSendFinishedFlag local uint8; TRUE parameter; FALSE parameter; SeatMemBtn input; DrMem_HeightHallPosi input; DrMem_LengthHallPosi input; DrMem_BackHallPosi input; DrMem_FrontHallPosi input; MemSetPC_Flag input; WaitTimer local uint8; CAL_DrMem_100MS parameter; PreMemSetStop input; MemSetStopReason output Enum: enMemStopCause; FLTempSeatMemSetSts local Enum: enMemSetFb; DrMem_AdjustEnable input; CAL_DrMem_90MS parameter; WaitTimeCnt local uint16

== stateflow chart Appl_DrMemory_CtrlModel/UpDataInputInfo/InputSignalProcess/MemoryRemindPreconditionDeal/MemoryRemindPrecondition/PosiCompareFunc/PosiCompareFunc ==
  (default) -> (junction 15)
  (junction 15) -> (junction 47) [order 1] : /* 没有记忆位置 */
      | [PosiReq == FALSE]
  (junction 15) -> (junction 17) [order 2]
  (junction 47) -> (junction 49) : /* 未记忆位置 */
      | {Result = 2;}
  (junction 17) -> (junction 19) [order 1] : /* 当前位置在记忆位置范围内 */
      | [CurrentH <= MemH + D_ToleranceDistance ...
      | && MemH <= CurrentH  + D_ToleranceDistance ...
      | && CurrentL <= MenL + D_ToleranceDistance ...
      | && MenL <= CurrentL  + D_ToleranceDistance ...
      | && CurrentB <= MemB + D_ToleranceDistance ...
      | && MemB <= CurrentB  + D_ToleranceDistance]
  (junction 17) -> (junction 23) [order 2] : {Result = FALSE;}
  (junction 19) -> (junction 21) : {Result = TRUE;}
  (junction 21) -> (junction 23)
  (junction 23) -> (junction 26)
  (junction 26) -> (junction 40) [order 1] : /* 8向调节 */
      | [AdjustEnable == 2]
  (junction 26) -> (junction 31) [order 2]
  (junction 40) -> (junction 42)
  (junction 42) -> (junction 33) [order 1] : /* 前部角度在位置 */
      | [CurrentF <= MemF + D_ToleranceDistance ...
      | && MemF <= CurrentF  + D_ToleranceDistance ...
      | && Result == TRUE]
  (junction 42) -> (junction 44) [order 2] : {Result = FALSE;}
  (junction 33) -> (junction 35) : {Result = TRUE;}
  (junction 44) -> (junction 31)
  (junction 35) -> (junction 44)
  (junction 49) -> (junction 35)
  (junction 31) -> (junction 38)
  data: MemH input uint16; MenL input uint16; MemB input uint16; MemF input uint16; CurrentH input uint16; CurrentL input uint16; CurrentB input uint16; CurrentF input uint16; Result output uint8; TRUE parameter; FALSE parameter; D_ToleranceDistance parameter; AdjustEnable input uint8; PosiReq input uint8

== stateflow chart Appl_DrMemory_CtrlModel/LogicCtrl/LocalAdjustCtrl/MemoryRemindLogic ==
  state SetCanSendEvent [function]
  state Out1 = GetCanSendEvent [function]
  state WriteFLSeatPosMsg(Sts) [function]
  state SetCanSendFLSeatPosMsg(In1) [function]
  state Init [commented out]
    en:
    FirstTimeCnt = 0;
    du:
    FirstTimeCnt += 1;
  state PositionNoChange [commented out]
    en:
    FLSeatPosMsg = FALSE;
    WriteFLSeatPosMsg(FLSeatPosMsg);
  state PositionNoChange1
    en:
    FLSeatPosMsg = FALSE;
  state PositionChange1
    en:
    FLSeatPosMsg = TRUE;
    SetCanSendFLSeatPosMsg(FLSeatPosMsg);
    SetCanSendEvent();
  state PositionChange [commented out]
    en:
    FLSeatPosMsg = TRUE;
    WriteFLSeatPosMsg(FLSeatPosMsg);
  (default) -> Init [commented out]
  (default) -> PositionNoChange1
  Init -> (junction 3) [commented out] : /* 上电获取eeprom延时 */
      | [FirstTimeCnt > CAL_DrMem_90MS]
  (junction 3) -> PositionNoChange [commented out]
  (junction 3) -> PositionChange [commented out] : /*FLSeatPosMsg存储的
      | EEPROM数据 == 0x1:enChange*/
      | [DrMem_FLSeatPosMsg == TRUE]
  PositionNoChange1 -> PositionChange1 : /*满足【前置条件】&&【触发条件1】
      | 运动类型由手动调节变为静止
      | && MemRemindPC_Flag == TRUE
      | &&(Result1st != TRUE
      | || Result2nd != TRUE
      | || Result3rd != TRUE)*/
      | [hasChangedFrom(DrMem_CurrentMoveType, ...
      | enSeatMotorRunType.EN_ManualEnable) ...
      | && DrMem_CurrentMoveType == enSeatMotorRunType.EN_NULL ...
      | && MemRemindPC_Flag == TRUE ...
      | && (Result1st != 2 || Result2nd != 2 || Result3rd != 2) ...
      | && Result1st != TRUE ...
      | && Result2nd != TRUE ...
      | && Result3rd != TRUE]
  PositionChange1 -> PositionNoChange1 [order 1] : /* 恢复出厂标志位 == TRUE 或前置条件不满足 */
      | [DrMem_GetRecoverDefaultFlag == TRUE ...
      | || MemRemindPC_Flag == FALSE]
  PositionChange1 -> PositionNoChange1 [order 2] : /* 快发时间超时 */
      | [GetCanSendEvent() == TRUE]
  PositionNoChange -> PositionChange [commented out] : /*满足【前置条件】&&【触发条件1】
      | 运动类型由手动调节变为静止
      | && MemRemindPC_Flag == TRUE
      | &&(Result1st != TRUE
      | || Result2nd != TRUE
      | || Result3rd != TRUE)*/
      | [hasChangedFrom(DrMem_CurrentMoveType, ...
      | enSeatMotorRunType.EN_ManualEnable) ...
      | && DrMem_CurrentMoveType == enSeatMotorRunType.EN_NULL ...
      | && MemRemindPC_Flag == TRUE ...
      | &&(Result1st != TRUE ...
      | && Result2nd != TRUE ...
      | && Result3rd != TRUE)]
  PositionChange -> PositionNoChange [commented out] : /*恢复出厂标志位 == TRUE */
      | [DrMem_GetRecoverDefaultFlag == TRUE]
  PositionChange -> PositionNoChange [commented out] : /*满足【前置条件】||【触发条件2】
      | (Result1st == TRUE
      | || Result2nd == TRUE
      | || Result3rd == TRUE)
      | || MemRemindPC_Flag == FALSE */
      | [(Result1st == TRUE ...
      | || Result2nd == TRUE ...
      | || Result3rd == TRUE) ...
      | || MemRemindPC_Flag == FALSE]
  data: Out1 function_output; Sts function_input; In1 function_input; FLSeatPosMsg output uint8; TRUE parameter; FALSE parameter; DrMem_FLSeatPosMsg input; MemRemindPC_Flag input; Result1st input; Result2nd input; Result3rd input; DrMem_CurrentMoveType input; DrMem_GetRecoverDefaultFlag input; FirstTimeCnt local uint8; CAL_DrMem_90MS parameter

== stateflow chart Appl_DrMemory_CtrlModel/UpDataInputInfo/InputSignalProcess/HmiMessageDeal/HmiDeal ==
  state MemoryMessageConflictDeal [parallel]
    settings: executionOrder=1
    (default) -> (junction 39)
    MemoryMessageConflictDeal -> (junction 39)
    (junction 39) -> (junction 43) : {ActionCnt = 0;}
    (junction 43) -> (junction 45) [order 1] : /* 调用1 */
        | [DrMem_IVI_FLSeatMemSet1 > enMemSet.EN_MemSet_NULL ...
        | && DrMem_IVI_FLSeatMemSet1 < enMemSet.EN_MemSet_Clean]
    (junction 43) -> (junction 47) [order 2]
    (junction 45) -> (junction 49) : {ActionCnt += 1;}
    (junction 49) -> (junction 47)
    (junction 47) -> (junction 231)
    (junction 231) -> (junction 233) [order 1] : /*调用2 */
        | [DrMem_IVI_FLSeatMemSet2 > enMemSet.EN_MemSet_NULL ...
        | &&DrMem_IVI_FLSeatMemSet2 < enMemSet.EN_MemSet_Clean]
    (junction 231) -> (junction 237) [order 2]
    (junction 233) -> (junction 235) : {ActionCnt += 1;}
    (junction 235) -> (junction 237)
    (junction 237) -> (junction 247)
    (junction 247) -> (junction 243) [order 1] : /* 调用3 */
        | [DrMem_IVI_FLSeatMemSet3 > enMemSet.EN_MemSet_NULL ...
        | &&DrMem_IVI_FLSeatMemSet3 < enMemSet.EN_MemSet_Clean]
    (junction 247) -> (junction 241) [order 2]
    (junction 243) -> (junction 242) : {ActionCnt += 1;}
    (junction 242) -> (junction 241)
    (junction 241) -> (junction 253)
    (junction 253) -> (junction 252) [order 1] : /* 存在冲突 */
        | [ActionCnt >= 2]
    (junction 253) -> (junction 257) [order 2] : {ActionFlag = TRUE;}
    (junction 252) -> (junction 251) : {ActionFlag = FALSE;}
    (junction 251) -> (junction 257)
    (junction 257) -> (junction 62)
  state AcquireMemoryButtonReq [parallel]
    settings: executionOrder=2
    state NoButtonConflict
      state FirstButton [parallel]
        settings: executionOrder=1
        (default) -> (junction 71)
        FirstButton -> (junction 71)
        (junction 71) -> (junction 74)
        (junction 74) -> (junction 76) [order 1] : /*   */
            | [DrMem_IVI_FLSeatMemSet1 == enMemSet.EN_MemSet_Mem]
        (junction 74) -> (junction 80) [order 2]
        (junction 76) -> (junction 78) : {SeatMemBtn = enMemBtn.EN_MemBtn_Set1;}
        (junction 78) -> (junction 80)
        (junction 80) -> (junction 84)
        (junction 84) -> (junction 86) [order 1] : /* 调用位置1 */
            | [DrMem_IVI_FLSeatMemSet1 == enMemSet.EN_MemSet_Call]
        (junction 84) -> (junction 90) [order 2]
        (junction 86) -> (junction 88) : {SeatMemBtn = enMemBtn.EN_MemBtn_Call1;}
        (junction 88) -> (junction 90)
        (junction 90) -> (junction 93)
        (junction 93) -> (junction 95) [commented out] : /* 清除位置1 */
            | [DrMem_IVI_FLSeatMemSet1 == enMemSet.EN_MemSet_Clean]
        (junction 93) -> (junction 99)
        (junction 95) -> (junction 97) [commented out] : {SeatMemBtn = enMemBtn.EN_MemBtn_Clear1;}
        (junction 97) -> (junction 99) [commented out]
        (junction 99) -> (junction 102)
      state SecondButton [parallel]
        settings: executionOrder=2
        (default) -> (junction 105)
        SecondButton -> (junction 105)
        (junction 105) -> (junction 110)
        (junction 110) -> (junction 114) [order 1] : /* 记忆位置2 */
            | [DrMem_IVI_FLSeatMemSet2 == enMemSet.EN_MemSet_Mem]
        (junction 110) -> (junction 117) [order 2]
        (junction 114) -> (junction 119) : {SeatMemBtn = enMemBtn.EN_MemBtn_Set2;}
        (junction 119) -> (junction 117)
        (junction 117) -> (junction 112)
        (junction 112) -> (junction 107) [order 1] : /* 调用位置2 */
            | [DrMem_IVI_FLSeatMemSet2 == enMemSet.EN_MemSet_Call]
        (junction 112) -> (junction 115) [order 2]
        (junction 107) -> (junction 120) : {SeatMemBtn = enMemBtn.EN_MemBtn_Call2;}
        (junction 120) -> (junction 115)
        (junction 115) -> (junction 125)
        (junction 125) -> (junction 126) [commented out] : /* 清除位置2 */
            | [DrMem_IVI_FLSeatMemSet2 == enMemSet.EN_MemSet_Clean]
        (junction 125) -> (junction 108)
        (junction 126) -> (junction 127) [commented out] : {SeatMemBtn = enMemBtn.EN_MemBtn_Clear2;}
        (junction 127) -> (junction 108) [commented out]
        (junction 108) -> (junction 128)
      state ThirdButton [parallel]
        settings: executionOrder=3
        (default) -> (junction 140)
        ThirdButton -> (junction 140)
        (junction 140) -> (junction 141)
        (junction 141) -> (junction 144) [order 1] : /* 记忆位置3 */
            | [DrMem_IVI_FLSeatMemSet3 == enMemSet.EN_MemSet_Mem]
        (junction 141) -> (junction 146) [order 2]
        (junction 144) -> (junction 147) : {SeatMemBtn = enMemBtn.EN_MemBtn_Set3;}
        (junction 147) -> (junction 146)
        (junction 146) -> (junction 150)
        (junction 150) -> (junction 153) [order 1] : /* 调用位置3 */
            | [DrMem_IVI_FLSeatMemSet3 == enMemSet.EN_MemSet_Call]
        (junction 150) -> (junction 155) [order 2]
        (junction 153) -> (junction 158) : {SeatMemBtn = enMemBtn.EN_MemBtn_Call3;}
        (junction 158) -> (junction 155)
        (junction 155) -> (junction 149)
        (junction 149) -> (junction 154) [commented out] : /* 清除位置3 */
            | [DrMem_IVI_FLSeatMemSet3 == enMemSet.EN_MemSet_Clean]
        (junction 149) -> (junction 145)
        (junction 154) -> (junction 138) [commented out] : {SeatMemBtn = enMemBtn.EN_MemBtn_Clear3;}
        (junction 138) -> (junction 145) [commented out]
        (junction 145) -> (junction 156)
      state CleanButtonReq [parallel]
        settings: executionOrder=4
        (default) -> (junction 172)
        CleanButtonReq -> (junction 172)
        (junction 172) -> (junction 175)
        (junction 175) -> (junction 177) [order 1] : /* 无记忆请求 */
            | [DrMem_IVI_FLSeatMemSet1 == enMemSet.EN_MemSet_NULL ...
            | && DrMem_IVI_FLSeatMemSet2 == enMemSet.EN_MemSet_NULL ...
            | && DrMem_IVI_FLSeatMemSet3 == enMemSet.EN_MemSet_NULL]
        (junction 175) -> (junction 181) [order 2]
        (junction 177) -> (junction 179) : {SeatMemBtn = enMemBtn.EN_MemBtn_NULL;}
        (junction 179) -> (junction 181)
        (junction 181) -> (junction 182)
    state ButtonConflict
      en:
      SeatMemBtn = enMemBtn.EN_MemBtn_NULL;
    (default) -> ButtonConflict
    ButtonConflict -> NoButtonConflict : /*无报文冲突*/
        | [ActionFlag == TRUE]
    NoButtonConflict -> ButtonConflict : /*报文冲突*/
        | [ActionFlag == FALSE]
  data: DrMem_IVI_FLSeatMemSet1 input; DrMem_IVI_FLSeatMemSet2 input; SeatMemBtn output Enum: enMemBtn; TRUE parameter; FALSE parameter; DrMem_IVI_FLSeatMemSet3 input; ActionFlag local double; ActionCnt local uint8
